simulink model "mcc"  (R2024a)
settings: Solver=VariableStepAuto  StartTime=0.0  StopTime=50  RelTol=1e-3
values from neighbouring files (symbols this model uses):
  A = zeros(2)    [parametrii.m]
  B = zeros(2)    [parametrii.m]
  C = zeros(2)    [parametrii.m]
  D = zeros(2)    [parametrii.m]
  k1 = 0.08    [parametrii.m]
  kE1 = 10    [parametrii.m]
  kE2 = 15    [parametrii.m]
  kem = 0.8    [parametrii.m]
  kEM = 0.02    [parametrii.m]
  kR = 5    [parametrii.m]
  kw = 1    [parametrii.m]
  T1 = 0.05    [parametrii.m]
  Ti = 0.1    [parametrii.m]
  Tr = 1    [parametrii.m]
  Tw = 0.5    [parametrii.m]
settings Model: Creator=paulhondola  LastModifiedBy=paulhondola

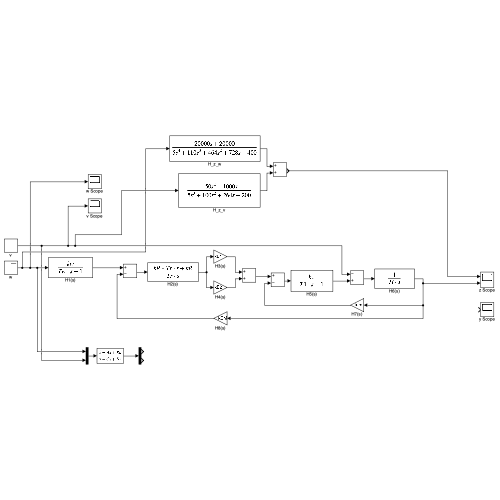
[thumbnail: Simulink's stored preview of the top-level diagram]
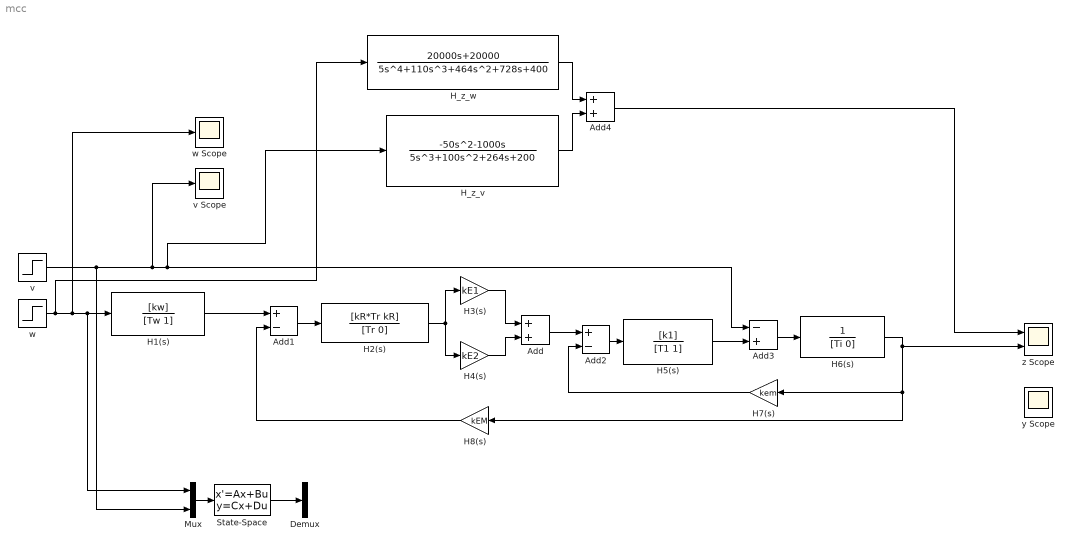
== system mcc ==
  Add : Sum
  Add1 : Sum  Inputs=+-
  Add2 : Sum  Inputs=+-
  Add3 : Sum  Inputs=-+
  Add4 : Sum
  Demux : Demux  Outputs=2
  H1(s) : TransferFcn  Numerator=[kw]  Denominator=[Tw 1]
  H2(s) : TransferFcn  Numerator=[kR*Tr kR]  Denominator=[Tr 0]
  H3(s) : Gain  Gain=kE1
  H4(s) : Gain  Gain=kE2
  H5(s) : TransferFcn  Numerator=[k1]  Denominator=[T1 1]
  H6(s) : TransferFcn  Denominator=[Ti 0]
  H7(s) : Gain  Gain=kem
  H8(s) : Gain  Gain=kEM
  H_z_v : TransferFcn  Numerator=[-50 -1000 0]  Denominator=[5 100 264 200]
  H_z_w : TransferFcn  Numerator=[20000 20000]  Denominator=[5 110 464 728 400]
  Mux : Mux  Inputs=2
  State-Space : StateSpace  A=A  B=B  C=C  D=D  InitialCondition=0
  v : Step  Time=25  SampleTime=0
  v Scope : Scope
  w : Step  Time=0  After=5  SampleTime=0
  w Scope : Scope
  y Scope : Scope
  z Scope : Scope  NumInputPorts=2
  wires:
  H2(s)/1 -> H4(s)/1, H3(s)/1
  H3(s)/1 -> Add/1
  H4(s)/1 -> Add/2
  w/1 -> Mux/1, H1(s)/1, w Scope/1, H_z_w/1
  Add1/1 -> H2(s)/1
  H1(s)/1 -> Add1/1
  Add/1 -> Add2/1
  v/1 -> Mux/2, v Scope/1, H_z_v/1, Add3/1
  H5(s)/1 -> Add3/2
  Add3/1 -> H6(s)/1
  H6(s)/1 -> H8(s)/1, H7(s)/1, z Scope/2
  H7(s)/1 -> Add2/2
  Add2/1 -> H5(s)/1
  H8(s)/1 -> Add1/2
  H_z_w/1 -> Add4/1
  H_z_v/1 -> Add4/2
  Mux/1 -> State-Space/1
  State-Space/1 -> Demux/1
  Add4/1 -> z Scope/1
